simulink model "AppSoftware"  (R2019a)
settings: Solver=FixedStepDiscrete  StartTime=0.0  StopTime=10  FixedStep=0.01  RelTol=1e-3  EnableMultiTasking=on
undefined symbols (not defined in the file): ADCResolutionmVproBit_C, AmbientLightOnTime_C, DebounceStepsToSetMinimumCurrError_C, IPROPFactor_C, IpropResistorValue_C, MaxMotorCurrent_C, MinMotorCurrent_C, sigbuilder_block
libraries: simulink x4
settings Model: DataDictionary=AppSoftware.sldd  EnableAccessToBaseWorkspace=off  Creator=The MathWorks, Inc.  LastModifiedBy=unix
settings DataIOCC: LimitDataPoints=on  ReturnWorkspaceOutputs=off
settings OptimizationCC: DefaultParameterBehavior=Inlined  PassReuseOutputArgsAs=Individual arguments  ZeroExternalMemoryAtStartup=off  ZeroInternalMemoryAtStartup=off  OptimizationLevel=level1  OptimizationCustomize=off
settings DebuggingCC: ParameterTunabilityLossMsg=error  AllowSymbolicDim=off  SFUnexpectedBacktrackingDiag=warning  SFNoUnconditionalDefaultTransitionDiag=warning  SFExecutionAtInitializationDiag=none  ArithmeticOperatorsInVariantConditions=warning
settings ModelReferenceCC: PropagateSignalLabelsOutOfModel=off
settings SFSimCC: SimUseLocalCustomCode=off  MATLABDynamicMemAlloc=off
settings RTWCC: SystemTargetFile=ert.tlc  GenCodeOnly=on  TemplateMakefile=ert_default_tmf  RTWUseLocalCustomCode=off  IncludeHyperlinkInReport=on
settings CodeAppCC: ForceParamTrailComments=on  IgnoreCustomStorageClasses=off  OperatorAnnotations=on  SimulinkDataObjDesc=on  SFDataObjDesc=on  InsertBlockDesc=on
settings ERTTargetCC: TargetLangStandard=C99 (ISO)  InlinedParameterPlacement=NonHierarchical  ERTCustomFileTemplate=example_file_process.tlc
settings ConfigComp: CovMetricSettings=dw  CovHtmlReporting=on  CovSaveCumulativeToWorkspaceVar=on  CovSaveSingleToWorkspaceVar=on  CovExternalEMLEnable=off

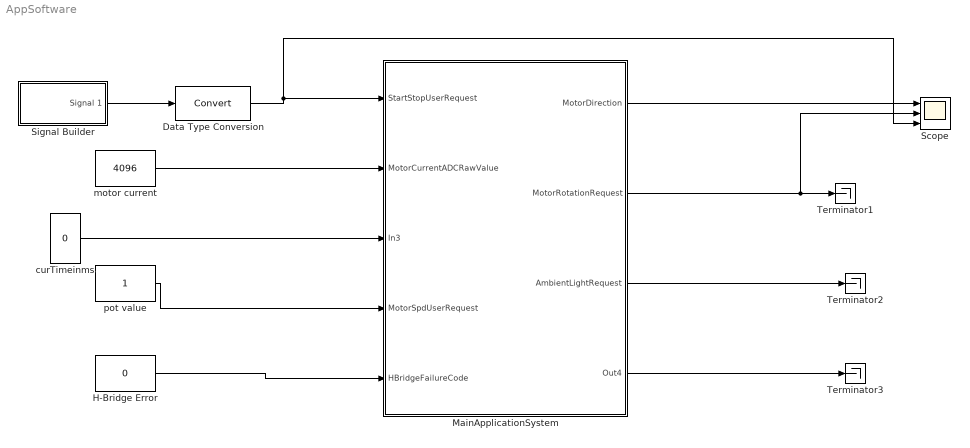
== system AppSoftware ==
  Data Type Conversion : DataTypeConversion
  H-Bridge Error : Constant  Value=0  OutDataTypeStr=Inherit: Inherit via back propagation
  MainApplicationSystem : Subsystem
  Scope : Scope  NumInputPorts=3
  Signal Builder : Subsystem  Tag=STV Subsys  LoadFcn=sigbuilder_block('load');  StartFcn=sigbuilder_block('start');  StopFcn=sigbuilder_block('stop');  ClipboardFcn=sigbuilder_block('clipboard');  mask(Sigbuilder block){tuvar=[0:10]}
      mask help: Simulink:masks:SigbuilderBlock_MD
      mask init:
      | if ~strcmp(get_param(bdroot(gcbh),'SimulationStatus'),'stopped') tuvar = sigbuilder_block('maskInit'); end
      settings: CopyFcn=sigbuilder_block('copy');  DeleteFcn=sigbuilder_block('delete');  ModelCloseFcn=sigbuilder_block('modelClose');  PreSaveFcn=sigbuilder_block('preSave');  PauseFcn=sigbuilder_block('pause');  ContinueFcn=sigbuilder_block('continue');  NameChangeFcn=sigbuilder_block('namechange');  OpenFcn=sigbuilder_block('open',[429.75 192 565.5 389.25 ]);  CloseFcn=sigbuilder_block('close');
      mask Display: plot(0, 0, 100, 100,[2, 2, 32, 32, 2], [68, 8, 8, 68, 68],[32, 2], [38, 38], [32, 19, 2],[53, 60, 44], [32, 17, 17, 2],[16, 16, 31, 31]);txt = getActiveGroup(gcbh);text(2, 100, txt,'verticalAlignment', 'top');
  Terminator1 : Terminator
  Terminator2 : Terminator
  Terminator3 : Terminator
  curTimeinms : Constant  Value=0  OutDataTypeStr=uint32
  motor current : Constant  Value=4096  OutDataTypeStr=Inherit: Inherit via back propagation
  pot value : Constant  OutDataTypeStr=Inherit: Inherit via back propagation
  wires:
  motor current/1 -> MainApplicationSystem/2(MotorCurrentADCRawValue)
  pot value/1 -> MainApplicationSystem/4(MotorSpdUserRequest)
  H-Bridge Error/1 -> MainApplicationSystem/5(HBridgeFailureCode)
  MainApplicationSystem/1(MotorDirection) -> Scope/1
  MainApplicationSystem/2(MotorRotationRequest) -> Scope/2, Terminator1/1
  MainApplicationSystem/3(AmbientLightRequest) -> Terminator2/1
  MainApplicationSystem/4(Out4) -> Terminator3/1
  Data Type Conversion/1 -> Scope/3, MainApplicationSystem/1(StartStopUserRequest)
  curTimeinms/1 -> MainApplicationSystem/3(In3)
  Signal Builder/1(Signal 1) -> Data Type Conversion/1

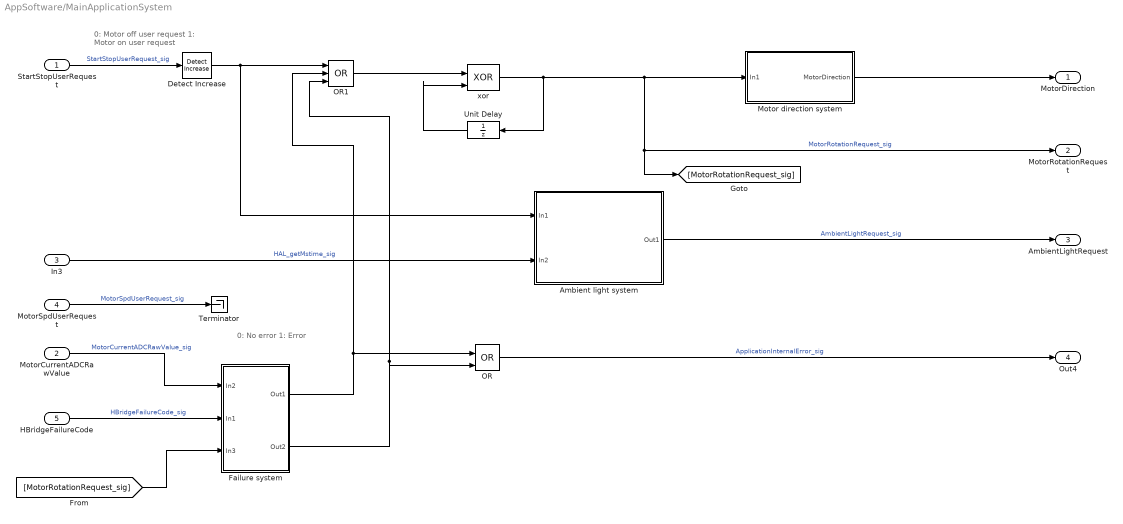
== system AppSoftware/MainApplicationSystem ==
  note: 0: No error
      | 1: Error
  note: 0: Motor off user request
      | 1: Motor on user request
  StartStopUserRequest : Inport
  MotorCurrentADCRawValue : Inport  Port=2
  In3 : Inport  Port=3
  MotorSpdUserRequest : Inport  Port=4
  HBridgeFailureCode : Inport  Port=5
  Ambient light system : Subsystem
  Detect Increase : simulink/Logic and Bit Operations/Detect Increase  vinit=0.0  OutDataTypeStr=boolean
  Failure system : Subsystem
  Motor direction system : Subsystem
  OR : Logic  Operator=OR  IconShape=distinctive  AllPortsSameDT=off  OutDataTypeStr=boolean
  OR1 : Logic  Operator=OR  Inputs=3  IconShape=distinctive  AllPortsSameDT=off  OutDataTypeStr=boolean
  Terminator : Terminator
  Unit Delay : UnitDelay  SampleTime=-1  HasFrameUpgradeWarning=on
  "xor " : Logic  Operator=XOR  IconShape=distinctive  AllPortsSameDT=off  OutDataTypeStr=boolean
  MotorDirection : Outport
  MotorRotationRequest : Outport  Port=2
  AmbientLightRequest : Outport  Port=3
  Out4 : Outport  Port=4
  wires:
  MotorCurrentADCRawValue/1 -> Failure system/1(In2)  "MotorCurrentADCRawValue_sig"
  "xor "/1 -> [MotorRotationRequest_sig], MotorRotationRequest/1, Motor direction system/1(In1), Unit Delay/1  "MotorRotationRequest_sig"
  Ambient light system/1(Out1) -> AmbientLightRequest/1  "AmbientLightRequest_sig"
  MotorSpdUserRequest/1 -> Terminator/1  "MotorSpdUserRequest_sig"
  StartStopUserRequest/1 -> Detect Increase/1  "StartStopUserRequest_sig"
  Unit Delay/1 -> "xor "/2
  HBridgeFailureCode/1 -> Failure system/2(In1)  "HBridgeFailureCode_sig"
  Motor direction system/1(MotorDirection) -> MotorDirection/1
  Detect Increase/1 -> OR1/1, Ambient light system/1(In1)
  [MotorRotationRequest_sig] -> Failure system/3(In3)
  In3/1 -> Ambient light system/2(In2)  "HAL_getMstime_sig"
  OR/1 -> Out4/1  "ApplicationInternalError_sig"
  OR1/1 -> "xor "/1
  Failure system/1(Out1) -> OR1/2, OR/1
  Failure system/2(Out2) -> OR1/3, OR/2

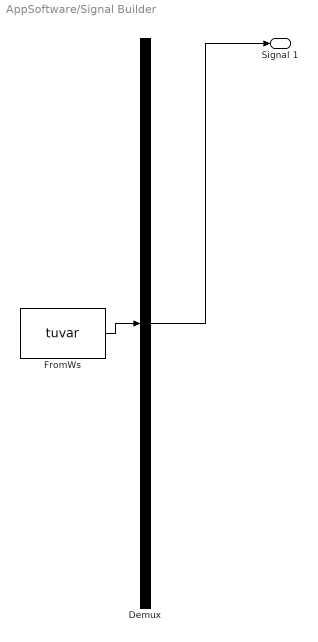
== system AppSoftware/Signal Builder ==
  Demux : Demux  Tag=STV Demux  Outputs=1
  FromWs : FromWorkspace  Tag=STV FromWs  VariableName=tuvar  SampleTime=0
      SigBuilderData=|
      | common.afterFinalStr = 'Extrapolate'
      | common.sampleTime = 0
      | dataSet.timeRange = [0 10]
      | dataSet.name = 'Group 1'
      | sbobj.Groups.Name = 'Group 1'
      | sbobj.Groups.Signals.Name = 'Signal 1'
      | sbobj.Groups.Signals.XData = [0 0.4 0.4 0.5 0.5 0.98 0.98 1.08 1.08 1.44 1.44 1.54 1.54 10]
      | sbobj.Groups.Signals.YData = [0 0 0.995 1 0 0 1 1 0 0 1 1 0 0]
  Signal 1 : Outport  Tag=STV Outport
  wires:
  Demux/1 -> Signal 1/1
  FromWs/1 -> Demux/1

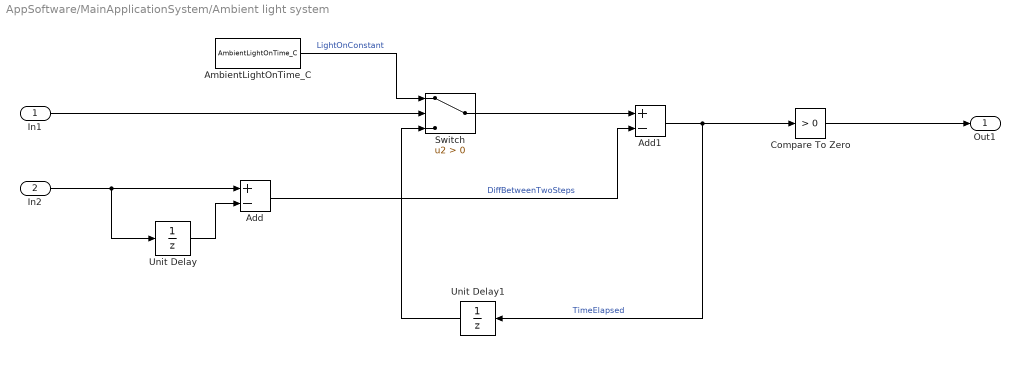
== system AppSoftware/MainApplicationSystem/Ambient light system ==
  In1 : Inport
  In2 : Inport  Port=2
  Add : Sum  Inputs=+-
  Add1 : Sum  Inputs=+-  SaturateOnIntegerOverflow=on
  AmbientLightOnTime_C : Constant  Value=AmbientLightOnTime_C  OutDataTypeStr=uint32
  Compare To Zero : simulink/Logic and Bit Operations/Compare To Zero  relop=>  OutDataTypeStr=boolean
  Switch : Switch  Criteria=u2 > Threshold
  Unit Delay : UnitDelay  SampleTime=-1  HasFrameUpgradeWarning=on
  Unit Delay1 : UnitDelay  InitialCondition=AmbientLightOnTime_C  SampleTime=-1  HasFrameUpgradeWarning=on
      settings: AttributesFormatString=%<InitialCondition>
  Out1 : Outport
  wires:
  In2/1 -> Add/1, Unit Delay/1
  Unit Delay/1 -> Add/2
  Add1/1 -> Compare To Zero/1, Unit Delay1/1  "TimeElapsed"
  Add/1 -> Add1/2  "DiffBetweenTwoSteps"
  Switch/1 -> Add1/1
  In1/1 -> Switch/2
  AmbientLightOnTime_C/1 -> Switch/1  "LightOnConstant"
  Unit Delay1/1 -> Switch/3
  Compare To Zero/1 -> Out1/1

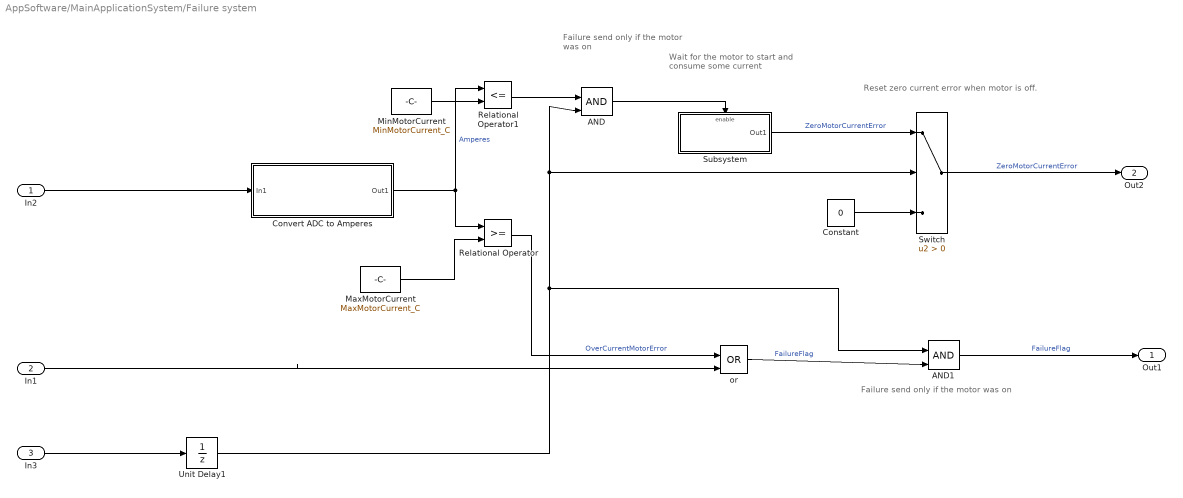
== system AppSoftware/MainApplicationSystem/Failure system ==
  note: Failure send only if the motor was on
  note: Reset zero current error when motor is off.
  note: Wait for the motor to start and consume some current
  note: Failure send only if the motor was on
  In2 : Inport
  In1 : Inport  Port=2
  In3 : Inport  Port=3
  AND : Logic  IconShape=distinctive  AllPortsSameDT=off  OutDataTypeStr=boolean
  AND1 : Logic  IconShape=distinctive  AllPortsSameDT=off  OutDataTypeStr=boolean
  Constant : Constant  Value=0  OutDataTypeStr=boolean
  Convert ADC to Amperes : Subsystem
  MaxMotorCurrent : Constant  Value=MaxMotorCurrent_C
  MinMotorCurrent : Constant  Value=MinMotorCurrent_C
  Relational Operator : RelationalOperator  OutDataTypeStr=boolean  InputSameDT=on
  Relational Operator1 : RelationalOperator  Operator=<=  OutDataTypeStr=boolean  InputSameDT=on
  Subsystem : Subsystem
  Switch : Switch  Criteria=u2 > Threshold
      settings: AttributesFormatString=|
      | Threshold = %<Threshold>
      | %<Criteria>
  Unit Delay1 : UnitDelay  SampleTime=-1  HasFrameUpgradeWarning=on
  or : Logic  Operator=OR  IconShape=distinctive  AllPortsSameDT=off  OutDataTypeStr=boolean
  Out1 : Outport
  Out2 : Outport  Port=2
  wires:
  MaxMotorCurrent/1 -> Relational Operator/2
  Relational Operator/1 -> or/1  "OverCurrentMotorError"
  In1/1 -> or/2
  AND1/1 -> Out1/1  "FailureFlag"
  MinMotorCurrent/1 -> Relational Operator1/2
  Switch/1 -> Out2/1  "ZeroMotorCurrentError"
  In3/1 -> Unit Delay1/1
  Unit Delay1/1 -> AND1/1, AND/2, Switch/2
  Relational Operator1/1 -> AND/1
  AND/1 -> Subsystem/Enable
  Subsystem/1(Out1) -> Switch/1  "ZeroMotorCurrentError"
  Constant/1 -> Switch/3
  Convert ADC to Amperes/1(Out1) -> Relational Operator/1, Relational Operator1/1  "Amperes"
  In2/1 -> Convert ADC to Amperes/1(In1)
  or/1 -> AND1/2  "FailureFlag"

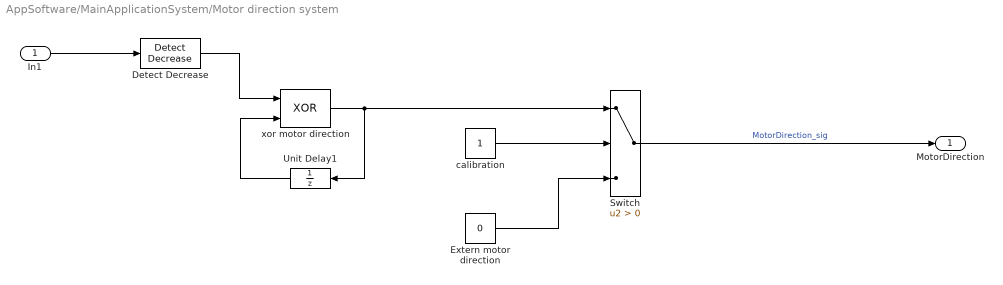
== system AppSoftware/MainApplicationSystem/Motor direction system ==
  In1 : Inport
  Detect Decrease : simulink/Logic and Bit Operations/Detect Decrease  vinit=0.0  OutDataTypeStr=boolean
  Extern motor direction : Constant  Value=0  OutDataTypeStr=boolean
  Switch : Switch  Criteria=u2 > Threshold
  Unit Delay1 : UnitDelay  SampleTime=-1  HasFrameUpgradeWarning=on
  "calibration " : Constant  OutDataTypeStr=boolean
  xor motor direction : Logic  Operator=XOR  IconShape=distinctive  AllPortsSameDT=off  OutDataTypeStr=boolean
  MotorDirection : Outport
  wires:
  Unit Delay1/1 -> xor motor direction/2
  In1/1 -> Detect Decrease/1
  Switch/1 -> MotorDirection/1  "MotorDirection_sig"
  Detect Decrease/1 -> xor motor direction/1
  xor motor direction/1 -> Unit Delay1/1, Switch/1
  Extern motor direction/1 -> Switch/3
  "calibration "/1 -> Switch/2

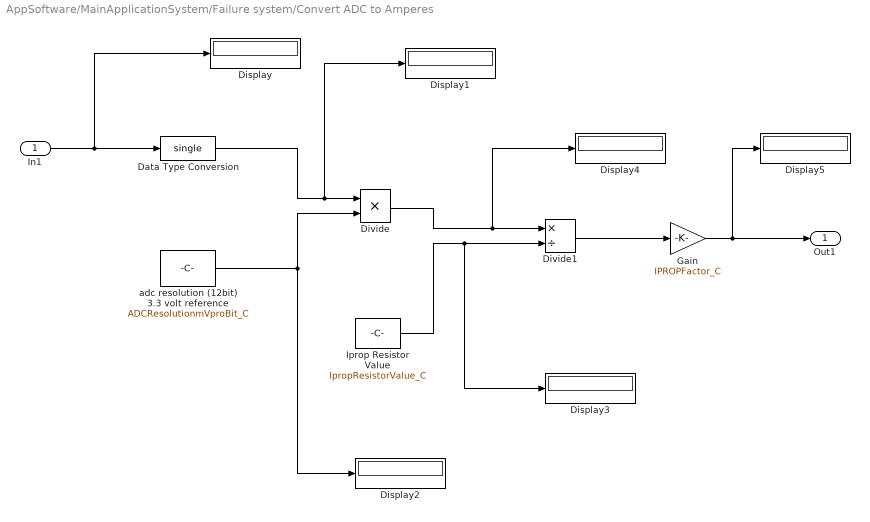
== system AppSoftware/MainApplicationSystem/Failure system/Convert ADC to Amperes ==
  In1 : Inport
  Data Type Conversion : DataTypeConversion  OutDataTypeStr=single
  Display{,1..5} (6 alike) : Display
  Divide : Product  Inputs=**
  Divide1 : Product  Inputs=*/
  Gain : Gain  Gain=IPROPFactor_C
  Iprop Resistor Value : Constant  Value=IpropResistorValue_C
  adc resolution (12bit) 3.3 volt reference : Constant  Value=ADCResolutionmVproBit_C  OutDataTypeStr=single
  Out1 : Outport
  wires:
  Divide1/1 -> Gain/1
  Gain/1 -> Display5/1, Out1/1
  adc resolution (12bit) 3.3 volt reference/1 -> Display2/1, Divide/2
  Data Type Conversion/1 -> Display1/1, Divide/1
  Iprop Resistor Value/1 -> Display3/1, Divide1/2
  In1/1 -> Display/1, Data Type Conversion/1
  Divide/1 -> Display4/1, Divide1/1

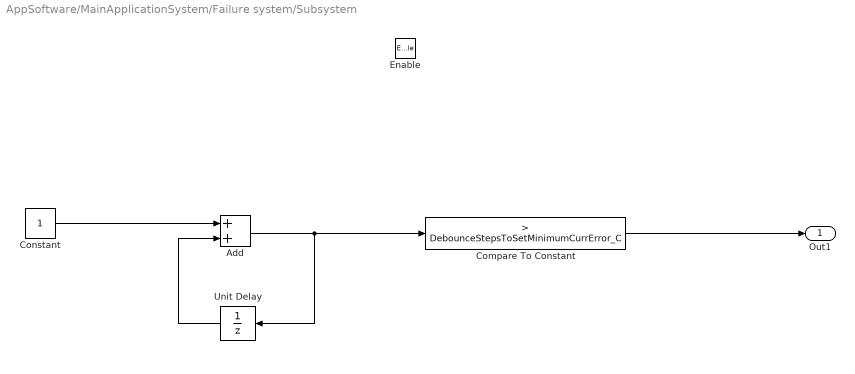
== system AppSoftware/MainApplicationSystem/Failure system/Subsystem ==
  Enable : EnablePort  StatesWhenEnabling=reset
  Add : Sum  SaturateOnIntegerOverflow=on
  Compare To Constant : simulink/Logic and Bit Operations/Compare To Constant  relop=>  const=DebounceStepsToSetMinimumCurrError_C  OutDataTypeStr=boolean
  Constant : Constant  OutDataTypeStr=uint8
  Unit Delay : UnitDelay  SampleTime=-1  HasFrameUpgradeWarning=on
      settings: AttributesFormatString=%<InitialCondition>
  Out1 : Outport
  wires:
  Constant/1 -> Add/1
  Add/1 -> Unit Delay/1, Compare To Constant/1
  Unit Delay/1 -> Add/2
  Compare To Constant/1 -> Out1/1
